simulink model "brake_mechanism_model"  (R2024b)
settings: Solver=ode4  StartTime=0.0  StopTime=5  FixedStep=0.05  RelTol=1e-3
settings Model: Creator=MrZang  LastModifiedBy=MrZang

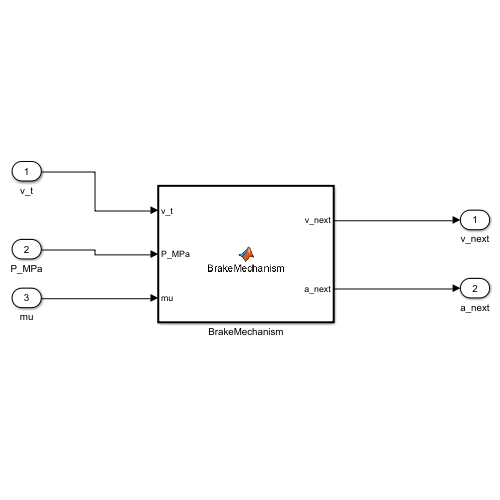
[thumbnail: Simulink's stored preview of the top-level diagram]
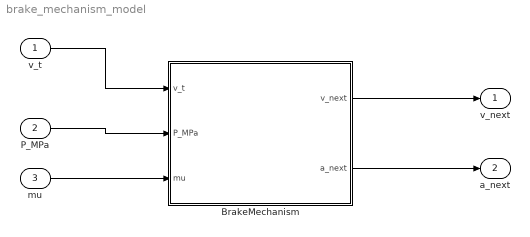
== system brake_mechanism_model ==
  v_t : Inport
  P_MPa : Inport  Port=2
  mu : Inport  Port=3
  BrakeMechanism : MATLAB Function  TreatAsAtomicUnit=on
  v_next : Outport
  a_next : Outport  Port=2
  wires:
  v_t/1 -> BrakeMechanism/1(v_t)
  P_MPa/1 -> BrakeMechanism/2(P_MPa)
  mu/1 -> BrakeMechanism/3(mu)
  BrakeMechanism/1(v_next) -> v_next/1
  BrakeMechanism/2(a_next) -> a_next/1

== matlab function brake_mechanism_model/BrakeMechanism ==
  data: v_t input; v_next output; P_MPa input; mu input; a_next output
function [v_next,a_next] = BrakeMechanism(v_t,P_MPa,mu)
%#codegen
m = 1800; g = 9.81; kBrake = 3500; dt = 0.05;
fBrake = max(P_MPa,0) * kBrake;
fMax = max(mu,0.01) * m * g;
fActual = min(fBrake, fMax);
a_next = -fActual / m;
v_next = max(v_t + a_next * dt, 0);
end
